simulink model "trocador_PS_PID_sim"  (R2020a)
settings: Solver=VariableStepAuto  StartTime=0.0  StopTime=tsim  MaxStep=0.01  RelTol=1e-3
values from neighbouring files (symbols this model uses):
  amppert = 0.5    [trocador_PS_PID.m]
  ampref = 1    [trocador_PS_PID.m]
  tpert = 50    [trocador_PS_PID.m]
  tref = 4    [trocador_PS_PID.m]
libraries: cstblocks x6
settings Model: Creator=treezao  LastModifiedBy=treezao

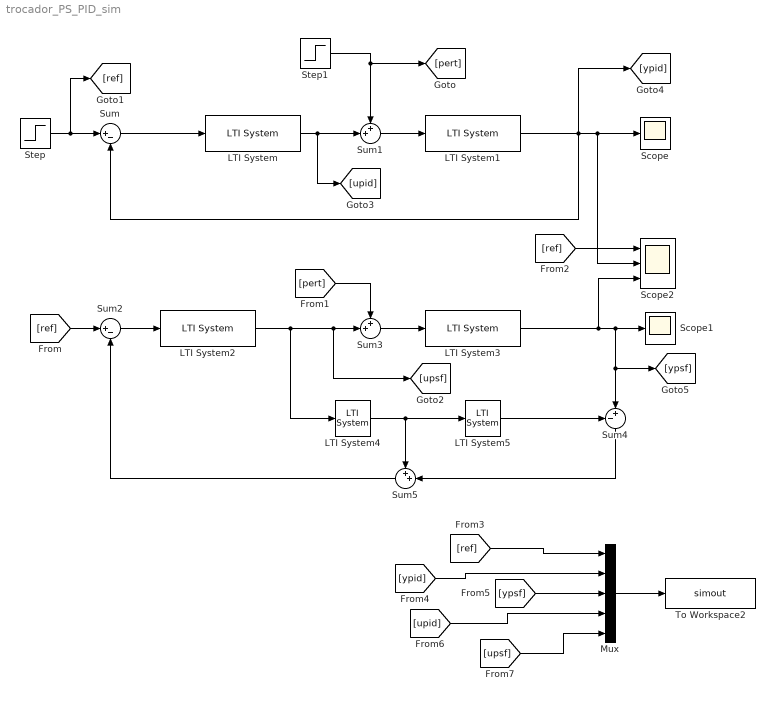
== system trocador_PS_PID_sim ==
  LTI System : cstblocks/LTI System  sys=Cz  IC=[]
  LTI System1 : cstblocks/LTI System  sys=P  IC=[]
  LTI System2 : cstblocks/LTI System  sys=Czps  IC=[]
  LTI System3 : cstblocks/LTI System  sys=P  IC=[]
  LTI System4 : cstblocks/LTI System  sys=Gnz  IC=[]
  LTI System5 : cstblocks/LTI System  sys=Lnz  IC=[]
  Mux : Mux  Inputs=5
  Scope : Scope
  Scope1 : Scope
  Scope2 : Scope  NumInputPorts=3
  Step : Step  Time=tref  After=ampref  SampleTime=0
  Step1 : Step  Time=tpert  After=amppert  SampleTime=0
  Sum : Sum  Inputs=|+-
  Sum1 : Sum  Inputs=++|
  Sum2 : Sum  Inputs=|+-
  Sum3 : Sum  Inputs=++|
  Sum4 : Sum  Inputs=-+|
  Sum5 : Sum  Inputs=++|
  To Workspace2 : ToWorkspace  VariableName=simout  SampleTime=-1
  wires:
  Step/1 -> [ref], Sum/1
  Sum/1 -> LTI System/1
  LTI System/1 -> [upid], Sum1/2
  Step1/1 -> [pert], Sum1/1
  Sum1/1 -> LTI System1/1
  LTI System1/1 -> [ypid], Sum/2, Scope2/2, Scope/1
  Sum2/1 -> LTI System2/1
  [ref] -> Sum2/1
  LTI System2/1 -> [upsf], Sum3/2, LTI System4/1
  Sum3/1 -> LTI System3/1
  LTI System3/1 -> Scope2/3, Scope1/1, [ypsf], Sum4/2
  [pert] -> Sum3/1
  LTI System4/1 -> Sum5/1, LTI System5/1
  LTI System5/1 -> Sum4/1
  Sum4/1 -> Sum5/2
  Sum5/1 -> Sum2/2
  [ref] -> Scope2/1
  Mux/1 -> To Workspace2/1
  [ref] -> Mux/1
  [ypid] -> Mux/2
  [ypsf] -> Mux/3
  [upid] -> Mux/4
  [upsf] -> Mux/5
